simulink model "SimulationDataInspector"  (R2015b)
settings: Solver=ode4  StartTime=5  StopTime=10  FixedStep=0.1  RelTol=1e-3
settings Model: Creator=LUBO  LastModifiedBy=LUBO
settings DataIOCC: InitialState=xFinal  LoadInitialState=on  SaveFinalState=on  SaveFormat=Array

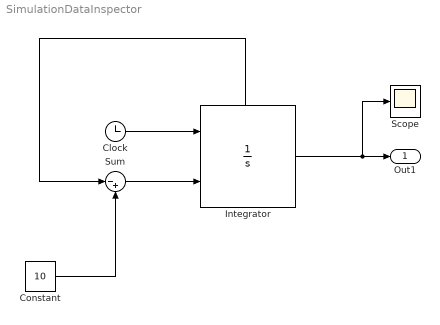
== system SimulationDataInspector ==
  Clock : Clock
  Constant : Constant  Value=10
  Integrator : Integrator  ExternalReset=falling  ShowStatePort=on
  Scope : Scope
  Sum : Sum  Inputs=|-+
  Out1 : Outport
  wires:
  Clock/1 -> Integrator/1
  Sum/1 -> Integrator/2
  Constant/1 -> Sum/2
  Integrator/1 -> Scope/1, Out1/1
  Integrator/State -> Sum/1
